simulink model "satellite_attitude_control_"  (R2023a)
settings: Solver=VariableStepAuto  StartTime=0.0  StopTime=300  FixedStep=0.001  MaxStep=0.001  RelTol=1e-3
libraries: slpidlib x2
settings Model: Creator=Mohamed Ezzelrgal  LastModifiedBy=Mohamed Ezzelrgal

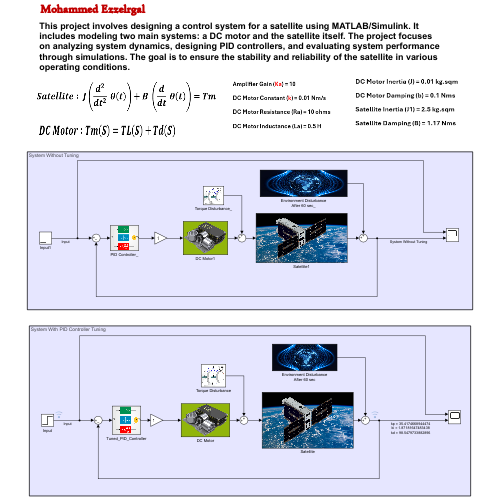
[thumbnail: Simulink's stored preview of the top-level diagram]
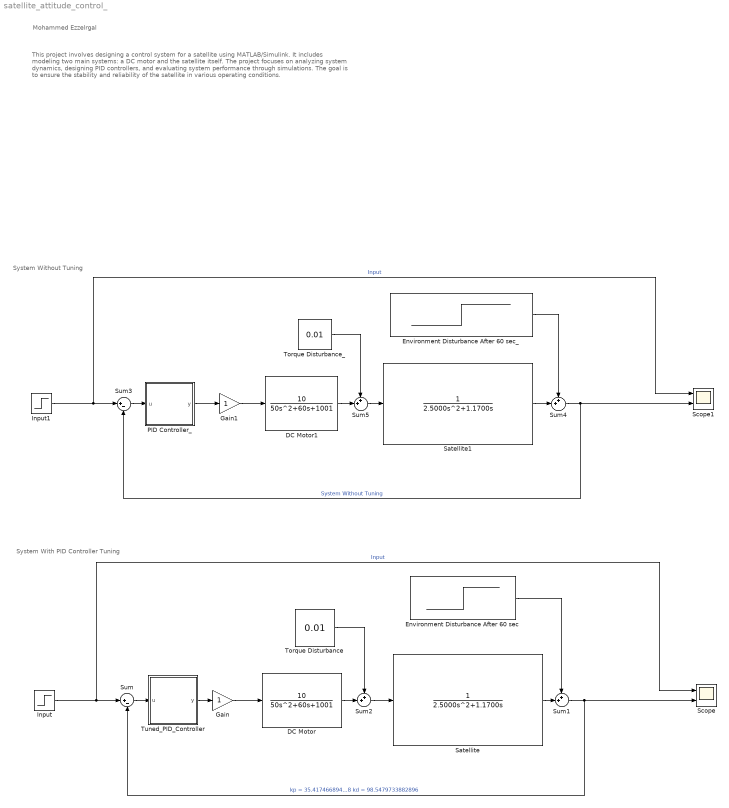
== system satellite_attitude_control_ ==
  note: This project involves designing a control system for a satellite using MATLAB/Simulink. It includes modeling two main systems: a DC motor and the satellite itself. The project focuses on analyzing system dynamics, designing PID controllers, and evaluating system performance through simulations. The goal is to ensure the stability and reliability of the satellite in various operating conditions.
  note: Mohammed Ezzelrgal
  note: System With PID Controller Tuning
  note: System Without Tuning
  DC Motor : TransferFcn  Numerator=[0 0 10]  Denominator=[50 60 1001]
      mask Display: image('C:\Users\User\Desktop\UKube-1_torque_reaction_drive_web (1).jpg'); % Use "Edit Image" on toolstrip to change.
  DC Motor1 : TransferFcn  Numerator=[0 0 10]  Denominator=[50 60 1001]
      mask Display: image('C:\Users\User\Desktop\UKube-1_torque_reaction_drive_web (1).jpg'); % Use "Edit Image" on toolstrip to change.
  Environment Disturbance After 60 sec : Step  Time=60  After=-0.4  SampleTime=0
      mask Display: image('C:\Users\User\Desktop\cd6c72bf29e9f773e06b8896d6927b79.jpg'); % Use "Edit Image" on toolstrip to change.
  Environment Disturbance After 60 sec_ : Step  Time=60  After=-0.4  SampleTime=0
      mask Display: image('C:\Users\User\Desktop\cd6c72bf29e9f773e06b8896d6927b79.jpg'); % Use "Edit Image" on toolstrip to change.
  Gain : Gain
  Gain1 : Gain
  Input : Step  SampleTime=0
  Input1 : Step  SampleTime=0
  PID Controller_ : Subsystem
      mask Display: image('C:\Users\User\Pictures\Screenshots\Screenshot 2024-04-15 103058.png'); % Use "Edit Image" on toolstrip to change.
  Satellite : TransferFcn  Numerator=[0 0 1]  Denominator=[2.5000 1.1700 0]
      mask Display: image('C:\Users\User\Desktop\EIVE-animiert.jpg'); % Use "Edit Image" on toolstrip to change.
  Satellite1 : TransferFcn  Numerator=[0 0 1]  Denominator=[2.5000 1.1700 0]
      mask Display: image('C:\Users\User\Desktop\EIVE-animiert.jpg'); % Use "Edit Image" on toolstrip to change.
  Scope : Scope  NumInputPorts=2
  Scope1 : Scope  NumInputPorts=2
  Sum : Sum  Inputs=|+-
  Sum{1..2,4..5} (4 alike) : Sum  Inputs=++|
  Sum3 : Sum  Inputs=|+-
  Torque Disturbance : Constant  Value=0.01
      mask Display: image('C:\Users\User\Pictures\Screenshots\Screenshot 2024-04-15 101415.png'); % Use "Edit Image" on toolstrip to change.
  Torque Disturbance_ : Constant  Value=0.01
      mask Display: image('C:\Users\User\Pictures\Screenshots\Screenshot 2024-04-15 101415.png'); % Use "Edit Image" on toolstrip to change.
  Tuned_PID_Controller : Subsystem
      mask Display: image('C:\Users\User\Pictures\Screenshots\Screenshot 2024-04-15 103058.png'); % Use "Edit Image" on toolstrip to change.
  wires:
  Input/1 -> Scope/1, Sum/1  "Input"
  Gain/1 -> DC Motor/1
  Torque Disturbance/1 -> Sum2/1
  DC Motor/1 -> Sum2/2
  Sum2/1 -> Satellite/1
  Satellite/1 -> Sum1/2
  Sum1/1 -> Scope/2, Sum/2  "kp = 35.4174668944474 ki = 1.87181647483438 kd = 98.5479733882896"
  Environment Disturbance After 60 sec/1 -> Sum1/1
  Environment Disturbance After 60 sec_/1 -> Sum4/1
  Sum4/1 -> Sum3/2, Scope1/2  "System Without Tuning"
  Satellite1/1 -> Sum4/2
  Sum5/1 -> Satellite1/1
  DC Motor1/1 -> Sum5/2
  Torque Disturbance_/1 -> Sum5/1
  Gain1/1 -> DC Motor1/1
  Input1/1 -> Sum3/1, Scope1/1  "Input"
  Sum3/1 -> PID Controller_/1(u)
  PID Controller_/1(y) -> Gain1/1
  Sum/1 -> Tuned_PID_Controller/1(u)
  Tuned_PID_Controller/1(y) -> Gain/1

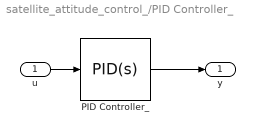
== system satellite_attitude_control_/PID Controller_ ==
  u : Inport
  PID Controller_ : slpidlib/PID Controller  Controller=PID  Form=Parallel  TimeDomain=Continuous-time  UseExternalTs=off  SampleTime=-1  IntegratorMethod=Forward Euler  FilterMethod=Forward Euler  ControllerParametersSource=internal  P=1  I=1  UseKiTs=off  D=0  N=100  UseFilter=on  TunerSelectOption=Transfer Function Based (PID Tuner App)  InitialConditionSource=internal  InitialConditionForIntegrator=0  InitialConditionForFilter=0  DifferentiatorICPrevScaledInput=0  ExternalReset=none  TrackingMode=off  Kt=1  LimitOutput=off  SatLimitsSource=internal  UpperSaturationLimit=inf  LowerSaturationLimit=-inf  LinearizeAsGain=on  AntiWindupMode=none  Kb=1  LimitIntegrator=off  UpperIntegratorSaturationLimit=inf  LowerIntegratorSaturationLimit=-inf  POutMin=[]  POutMax=[]  IOutMin=[]  IOutMax=[]  DOutMin=[]  DOutMax=[]  NOutMin=[]  NOutMax=[]  SumOutMin=[]  SumOutMax=[]  SaturationOutMin=[]  SaturationOutMax=[]  PParamMin=[]  PParamMax=[]  IParamMin=[]  IParamMax=[]  DParamMin=[]  DParamMax=[]  NParamMin=[]  NParamMax=[]  KbParamMin=[]  KbParamMax=[]  KtParamMin=[]  KtParamMax=[]  KbOutMin=[]  KbOutMax=[]  KtOutMin=[]  KtOutMax=[]  IntegratorOutMin=[]  IntegratorOutMax=[]  FilterOutMin=[]  FilterOutMax=[]  SumI1OutMin=[]  SumI1OutMax=[]  SumI2OutMin=[]  SumI2OutMax=[]  SumI3OutMin=[]  SumI3OutMax=[]  SumI4OutMin=[]  SumI4OutMax=[]  SumDOutMin=[]  SumDOutMax=[]  DifferentiatorOutMin=[]  DifferentiatorOutMax=[]  FilterDiffOutCoefMin=[]  FilterDiffOutCoefMax=[]  ReciprocalOutMin=[]  ReciprocalOutMax=[]  SumDenOutMin=[]  SumDenOutMax=[]  SumNumOutMin=[]  SumNumOutMax=[]  DivideOutMin=[]  DivideOutMax=[]  UdiffTsProdOutMin=[]  UdiffTsProdOutMax=[]  NTsProdOutMin=[]  NTsProdOutMax=[]  UintegralTsProdOutMin=[]  UintegralTsProdOutMax=[]  UngainTsProdOutMin=[]  UngainTsProdOutMax=[]  ClampingZeroOutDataTypeStr=Inherit: Inherit via back propagation  ClampingZeroOutMin=[]  ClampingZeroOutMax=[]  FilterDenConstantOutDataTypeStr=Inherit: Inherit via back propagation  FilterDenConstantOutMin=[]  FilterDenConstantOutMax=[]  PCopyOutDataTypeStr=Inherit: Inherit via back propagation  PCopyOutMin=[]  PCopyOutMax=[]  NCopyOutDataTypeStr=Inherit: Inherit via back propagation  NCopyOutMin=[]  NCopyOutMax=[]  IntegratorContinuousStateAttributes=''  IntegratorStateMustResolveToSignalObject=off  IntegratorRTWStateStorageClass=Auto  FilterContinuousStateAttributes=''  FilterStateMustResolveToSignalObject=off  FilterRTWStateStorageClass=Auto  ParallelPVariant=InternalParameters  IdealPVariant=Disabled  IVariant=InternalParameters  DVariant=InternalParameters  IntegratorVariant=Continuous  SatVariant=Disabled  AWVariant=Passthrough  PCopyVariant=Disabled  TRVariant=Disabled  FdbkBlocksVariant=Forward  IdealPFdbkVariant=Disabled  SatFdbkVariant=Disabled  DerivativeFilterVariant=ContFilter  NVariant=InternalParameters  NCopyVariant=Disabled  FilterICVariant=InternalICsFilter  IntegratorICVariant=InternalICs  ExternalResetVariant=Disabled  TRSumVariant=Passthrough  SumFdbkVariant=Disabled  SumVariant=Sum_PID  TsampFilterVariant=InternalTs  TsampNgainVariant=Passthrough  TsampIntegralVariant=Disabled_SignalSpec  ExternalSaturationOutDataTypeStr=Inherit: Same as second input
  y : Outport
  wires:
  PID Controller_/1 -> y/1
  u/1 -> PID Controller_/1

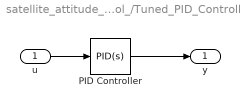
== system satellite_attitude_control_/Tuned_PID_Controller ==
  u : Inport
  PID Controller : slpidlib/PID Controller  Controller=PID  Form=Parallel  TimeDomain=Continuous-time  UseExternalTs=off  SampleTime=-1  IntegratorMethod=Forward Euler  FilterMethod=Forward Euler  ControllerParametersSource=internal  P=35.4174668944474  I=1.87181647483438  UseKiTs=off  D=98.5479733882896  N=1.30017780980392  UseFilter=on  TunerSelectOption=Transfer Function Based (PID Tuner App)  InitialConditionSource=internal  InitialConditionForIntegrator=0  InitialConditionForFilter=0  DifferentiatorICPrevScaledInput=0  ExternalReset=none  TrackingMode=off  Kt=1  LimitOutput=off  SatLimitsSource=internal  UpperSaturationLimit=inf  LowerSaturationLimit=-inf  LinearizeAsGain=on  AntiWindupMode=none  Kb=1  LimitIntegrator=off  UpperIntegratorSaturationLimit=inf  LowerIntegratorSaturationLimit=-inf  POutMin=[]  POutMax=[]  IOutMin=[]  IOutMax=[]  DOutMin=[]  DOutMax=[]  NOutMin=[]  NOutMax=[]  SumOutMin=[]  SumOutMax=[]  SaturationOutMin=[]  SaturationOutMax=[]  PParamMin=[]  PParamMax=[]  IParamMin=[]  IParamMax=[]  DParamMin=[]  DParamMax=[]  NParamMin=[]  NParamMax=[]  KbParamMin=[]  KbParamMax=[]  KtParamMin=[]  KtParamMax=[]  KbOutMin=[]  KbOutMax=[]  KtOutMin=[]  KtOutMax=[]  IntegratorOutMin=[]  IntegratorOutMax=[]  FilterOutMin=[]  FilterOutMax=[]  SumI1OutMin=[]  SumI1OutMax=[]  SumI2OutMin=[]  SumI2OutMax=[]  SumI3OutMin=[]  SumI3OutMax=[]  SumI4OutMin=[]  SumI4OutMax=[]  SumDOutMin=[]  SumDOutMax=[]  DifferentiatorOutMin=[]  DifferentiatorOutMax=[]  FilterDiffOutCoefMin=[]  FilterDiffOutCoefMax=[]  ReciprocalOutMin=[]  ReciprocalOutMax=[]  SumDenOutMin=[]  SumDenOutMax=[]  SumNumOutMin=[]  SumNumOutMax=[]  DivideOutMin=[]  DivideOutMax=[]  UdiffTsProdOutMin=[]  UdiffTsProdOutMax=[]  NTsProdOutMin=[]  NTsProdOutMax=[]  UintegralTsProdOutMin=[]  UintegralTsProdOutMax=[]  UngainTsProdOutMin=[]  UngainTsProdOutMax=[]  ClampingZeroOutDataTypeStr=Inherit: Inherit via back propagation  ClampingZeroOutMin=[]  ClampingZeroOutMax=[]  FilterDenConstantOutDataTypeStr=Inherit: Inherit via back propagation  FilterDenConstantOutMin=[]  FilterDenConstantOutMax=[]  PCopyOutDataTypeStr=Inherit: Inherit via back propagation  PCopyOutMin=[]  PCopyOutMax=[]  NCopyOutDataTypeStr=Inherit: Inherit via back propagation  NCopyOutMin=[]  NCopyOutMax=[]  IntegratorContinuousStateAttributes=''  IntegratorStateMustResolveToSignalObject=off  IntegratorRTWStateStorageClass=Auto  FilterContinuousStateAttributes=''  FilterStateMustResolveToSignalObject=off  FilterRTWStateStorageClass=Auto  ParallelPVariant=InternalParameters  IdealPVariant=Disabled  IVariant=InternalParameters  DVariant=InternalParameters  IntegratorVariant=Continuous  SatVariant=Disabled  AWVariant=Passthrough  PCopyVariant=Disabled  TRVariant=Disabled  FdbkBlocksVariant=Forward  IdealPFdbkVariant=Disabled  SatFdbkVariant=Disabled  DerivativeFilterVariant=ContFilter  NVariant=InternalParameters  NCopyVariant=Disabled  FilterICVariant=InternalICsFilter  IntegratorICVariant=InternalICs  ExternalResetVariant=Disabled  TRSumVariant=Passthrough  SumFdbkVariant=Disabled  SumVariant=Sum_PID  TsampFilterVariant=InternalTs  TsampNgainVariant=Passthrough  TsampIntegralVariant=Disabled_SignalSpec  ExternalSaturationOutDataTypeStr=Inherit: Same as second input
  y : Outport
  wires:
  u/1 -> PID Controller/1
  PID Controller/1 -> y/1
